simulink model "HybridController"  (Simulink 7.7)
settings: Solver=ode45  StartTime=0.0  StopTime=10.0  RelTol=1e-3
undefined symbols (not defined in the file): sigbuilder_block
settings Model: Creator=META-DEMO  LastModifiedBy=META-DEMO

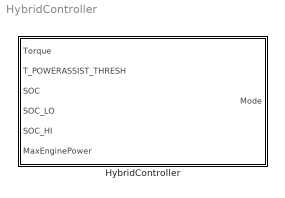
== system HybridController ==
  HybridController : Subsystem

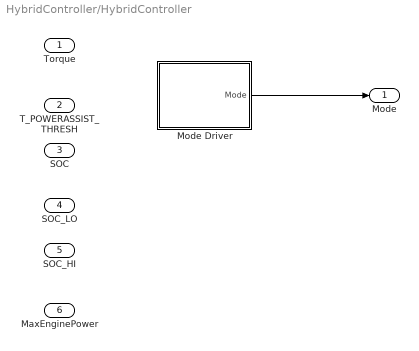
== system HybridController/HybridController ==
  Torque : Inport
  T_POWERASSIST_THRESH : Inport  Port=2
  SOC : Inport  Port=3
  SOC_LO : Inport  Port=4
  SOC_HI : Inport  Port=5
  MaxEnginePower : Inport  Port=6
  Mode Driver : Subsystem  Tag=STV Subsys  LoadFcn=sigbuilder_block('load');  StartFcn=sigbuilder_block('start');  StopFcn=sigbuilder_block('stop');  ClipboardFcn=sigbuilder_block('clipboard');  mask(Sigbuilder block){}
      mask help: Create and generate interchangeable groups of signals whose waveforms are piecewise linear.
      mask init:
      | if ~strcmp(get_param(bdroot(gcbh),'SimulationStatus'),'stopped') tuvar = sigbuilder_block('maskInit'); end
      settings: CopyFcn=sigbuilder_block('copy');  DeleteFcn=sigbuilder_block('delete');  ModelCloseFcn=sigbuilder_block('modelClose');  PreSaveFcn=sigbuilder_block('preSave');  NameChangeFcn=sigbuilder_block('namechange');  OpenFcn=sigbuilder_block('open',[164.483 25.4483 970.138 502.759 ]);  CloseFcn=sigbuilder_block('close');
      mask Display: plot(0,0,100,100,[10,10,40,40,10],[80,20,20,80,80],[40,10],[50,50], [40,27,10],[65,72,56],[40,25,25,10],[28,28,43,43]);
  Mode : Outport
  wires:
  Mode Driver/1(Mode) -> Mode/1

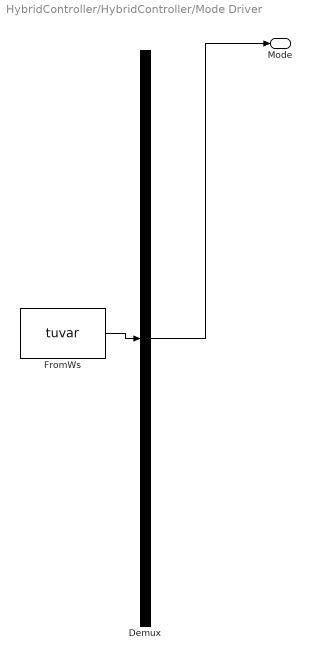
== system HybridController/HybridController/Mode Driver ==
  Demux : Demux  Tag=STV Demux  Outputs=1
  FromWs : FromWorkspace  Tag=STV FromWs  VariableName=tuvar  SampleTime=0  SigBuilderData=DataTag0  VnvData=DataTag1
      SigBuilderData=|
      | common.afterFinalStr = 'Extrapolate'
      | common.sampleTime = 0
      | dataSet.timeRange = [0 100]
      | dataSet.name = 'Group 1'
      | sbobj.Groups.Name = 'Group 1'
      | sbobj.Groups.Signals.Name = 'Mode'
      | sbobj.Groups.Signals.XData = [0 10 10 36.8 36.8 70 70 90 90 100]
      | sbobj.Groups.Signals.YData = [2 2 0 0 1 1 0 0 2 2]
  Mode : Outport  Tag=STV Outport
  wires:
  Demux/1 -> Mode/1
  FromWs/1 -> Demux/1
